simulink model "sampleModel1488"  (R2023a)
settings: Solver=VariableStepAuto  StartTime=0.0  StopTime=10.0  RelTol=1e-3
undefined symbols (not defined in the file): b011101a, b0c8, bf87616c, DiscIntNeverNeededParam, Newton, Raphson
libraries: simulink x171, slpidlib x32, simulink_need_slupdate x2
(part 6 of 6)

== system sampleModel1488/cfblk166/cfblk10 ==
  cfblk1 : Inport
  cfblk13 : Inport  Port=2
  cfblk14 : Inport  Port=3
  cfblk15 : Inport  Port=4
  cfblk10 : PermuteDimensions
  cfblk11 : Rounding
  cfblk12 : Sum  Inputs=|++
  cfblk3 : slpidlib/PID Controller (2DOF)  Controller=PID  Form=Parallel  TimeDomain=Discrete-time  UseExternalTs=off  SampleTime=1  IntegratorMethod=Forward Euler  FilterMethod=Forward Euler  ControllerParametersSource=internal  P=1  I=1  UseKiTs=off  D=0  N=100  UseFilter=on  b=1  c=1  TunerSelectOption=Transfer Function Based (PID Tuner App)  InitialConditionSource=internal  InitialConditionForIntegrator=0  InitialConditionForFilter=0  DifferentiatorICPrevScaledInput=0  ExternalReset=none  TrackingMode=off  Kt=1  LimitOutput=off  SatLimitsSource=internal  UpperSaturationLimit=inf  LowerSaturationLimit=-inf  LinearizeAsGain=off  AntiWindupMode=none  Kb=1  LimitIntegrator=off  UpperIntegratorSaturationLimit=inf  LowerIntegratorSaturationLimit=-inf  POutMin=[]  POutMax=[]  IOutMin=[]  IOutMax=[]  DOutMin=[]  DOutMax=[]  NOutMin=[]  NOutMax=[]  bOutMin=[]  bOutMax=[]  cOutMin=[]  cOutMax=[]  SumOutMin=[]  SumOutMax=[]  SaturationOutMin=[]  SaturationOutMax=[]  PParamMin=[]  PParamMax=[]  IParamMin=[]  IParamMax=[]  DParamMin=[]  DParamMax=[]  NParamMin=[]  NParamMax=[]  bParamMin=[]  bParamMax=[]  cParamMin=[]  cParamMax=[]  KbParamMin=[]  KbParamMax=[]  KtParamMin=[]  KtParamMax=[]  KbOutMin=[]  KbOutMax=[]  KtOutMin=[]  KtOutMax=[]  IntegratorOutMin=[]  IntegratorOutMax=[]  FilterOutMin=[]  FilterOutMax=[]  SumI1OutMin=[]  SumI1OutMax=[]  SumI2OutMin=[]  SumI2OutMax=[]  SumI3OutMin=[]  SumI3OutMax=[]  SumI4OutMin=[]  SumI4OutMax=[]  SumDOutMin=[]  SumDOutMax=[]  Sum1OutMin=[]  Sum1OutMax=[]  Sum2OutMin=[]  Sum2OutMax=[]  Sum3OutMin=[]  Sum3OutMax=[]  DifferentiatorOutMin=[]  DifferentiatorOutMax=[]  FilterDiffOutCoefMin=[]  FilterDiffOutCoefMax=[]  ReciprocalOutMin=[]  ReciprocalOutMax=[]  SumDenOutMin=[]  SumDenOutMax=[]  SumNumOutMin=[]  SumNumOutMax=[]  DivideOutMin=[]  DivideOutMax=[]  UdiffTsProdOutMin=[]  UdiffTsProdOutMax=[]  NTsProdOutMin=[]  NTsProdOutMax=[]  UintegralTsProdOutMin=[]  UintegralTsProdOutMax=[]  UngainTsProdOutMin=[]  UngainTsProdOutMax=[]  ClampingZeroOutDataTypeStr=Inherit: Inherit via back propagation  ClampingZeroOutMin=[]  ClampingZeroOutMax=[]  FilterDenConstantOutDataTypeStr=Inherit: Inherit via back propagation  FilterDenConstantOutMin=[]  FilterDenConstantOutMax=[]  PCopyOutDataTypeStr=Inherit: Inherit via back propagation  PCopyOutMin=[]  PCopyOutMax=[]  NCopyOutDataTypeStr=Inherit: Inherit via back propagation  NCopyOutMin=[]  NCopyOutMax=[]  IntegratorContinuousStateAttributes=''  IntegratorStateMustResolveToSignalObject=off  IntegratorRTWStateStorageClass=Auto  FilterContinuousStateAttributes=''  FilterStateMustResolveToSignalObject=off  FilterRTWStateStorageClass=Auto  ParallelPVariant=InternalParameters  IdealPVariant=Disabled  IVariant=InternalParameters  DVariant=InternalParameters  bVariant=InternalParameters  cVariant=InternalParameters  IntegratorVariant=Discrete  SatVariant=Disabled  AWVariant=Passthrough  PCopyVariant=Disabled  TRVariant=Disabled  FdbkBlocksVariant=Forward  IdealPFdbkVariant=Disabled  SatFdbkVariant=Disabled  DerivativeFilterVariant=ForwardEulerFilter  NVariant=InternalParameters  NCopyVariant=Disabled  FilterICVariant=InternalICsFilter  IntegratorICVariant=InternalICs  ExternalResetVariant=Disabled  TRSumVariant=Passthrough  SumFdbkVariant=Disabled  SumVariant=Sum_PID  TsampFilterVariant=InternalTs  TsampNgainVariant=Passthrough  TsampIntegralVariant=Disabled_SignalSpec  ExternalSaturationOutDataTypeStr=Inherit: Same as second input
      settings: LibrarySourceBlock=simulink/Discrete/Discrete PID Controller (2DOF)
  cfblk4 : DiscreteZeroPole  Poles=[0 0.5]  Gain=1
  cfblk5 : DiscreteZeroPole  Poles=[0 0.5]  Gain=1
  cfblk6 : slpidlib/PID Controller  Controller=PID  Form=Parallel  TimeDomain=Discrete-time  UseExternalTs=off  SampleTime=1  IntegratorMethod=Forward Euler  FilterMethod=Forward Euler  ControllerParametersSource=internal  P=1  I=1  UseKiTs=off  D=0  N=100  UseFilter=on  TunerSelectOption=Transfer Function Based (PID Tuner App)  InitialConditionSource=internal  InitialConditionForIntegrator=0  InitialConditionForFilter=0  DifferentiatorICPrevScaledInput=0  ExternalReset=none  TrackingMode=off  Kt=1  LimitOutput=off  SatLimitsSource=internal  UpperSaturationLimit=inf  LowerSaturationLimit=-inf  LinearizeAsGain=off  AntiWindupMode=none  Kb=1  LimitIntegrator=off  UpperIntegratorSaturationLimit=inf  LowerIntegratorSaturationLimit=-inf  POutMin=[]  POutMax=[]  IOutMin=[]  IOutMax=[]  DOutMin=[]  DOutMax=[]  NOutMin=[]  NOutMax=[]  SumOutMin=[]  SumOutMax=[]  SaturationOutMin=[]  SaturationOutMax=[]  PParamMin=[]  PParamMax=[]  IParamMin=[]  IParamMax=[]  DParamMin=[]  DParamMax=[]  NParamMin=[]  NParamMax=[]  KbParamMin=[]  KbParamMax=[]  KtParamMin=[]  KtParamMax=[]  KbOutMin=[]  KbOutMax=[]  KtOutMin=[]  KtOutMax=[]  IntegratorOutMin=[]  IntegratorOutMax=[]  FilterOutMin=[]  FilterOutMax=[]  SumI1OutMin=[]  SumI1OutMax=[]  SumI2OutMin=[]  SumI2OutMax=[]  SumI3OutMin=[]  SumI3OutMax=[]  SumI4OutMin=[]  SumI4OutMax=[]  SumDOutMin=[]  SumDOutMax=[]  DifferentiatorOutMin=[]  DifferentiatorOutMax=[]  FilterDiffOutCoefMin=[]  FilterDiffOutCoefMax=[]  ReciprocalOutMin=[]  ReciprocalOutMax=[]  SumDenOutMin=[]  SumDenOutMax=[]  SumNumOutMin=[]  SumNumOutMax=[]  DivideOutMin=[]  DivideOutMax=[]  UdiffTsProdOutMin=[]  UdiffTsProdOutMax=[]  NTsProdOutMin=[]  NTsProdOutMax=[]  UintegralTsProdOutMin=[]  UintegralTsProdOutMax=[]  UngainTsProdOutMin=[]  UngainTsProdOutMax=[]  ClampingZeroOutDataTypeStr=Inherit: Inherit via back propagation  ClampingZeroOutMin=[]  ClampingZeroOutMax=[]  FilterDenConstantOutDataTypeStr=Inherit: Inherit via back propagation  FilterDenConstantOutMin=[]  FilterDenConstantOutMax=[]  PCopyOutDataTypeStr=Inherit: Inherit via back propagation  PCopyOutMin=[]  PCopyOutMax=[]  NCopyOutDataTypeStr=Inherit: Inherit via back propagation  NCopyOutMin=[]  NCopyOutMax=[]  IntegratorContinuousStateAttributes=''  IntegratorStateMustResolveToSignalObject=off  IntegratorRTWStateStorageClass=Auto  FilterContinuousStateAttributes=''  FilterStateMustResolveToSignalObject=off  FilterRTWStateStorageClass=Auto  ParallelPVariant=InternalParameters  IdealPVariant=Disabled  IVariant=InternalParameters  DVariant=InternalParameters  IntegratorVariant=Discrete  SatVariant=Disabled  AWVariant=Passthrough  PCopyVariant=Disabled  TRVariant=Disabled  FdbkBlocksVariant=Forward  IdealPFdbkVariant=Disabled  SatFdbkVariant=Disabled  DerivativeFilterVariant=ForwardEulerFilter  NVariant=InternalParameters  NCopyVariant=Disabled  FilterICVariant=InternalICsFilter  IntegratorICVariant=InternalICs  ExternalResetVariant=Disabled  TRSumVariant=Passthrough  SumFdbkVariant=Disabled  SumVariant=Sum_PID  TsampFilterVariant=InternalTs  TsampNgainVariant=Passthrough  TsampIntegralVariant=Disabled_SignalSpec  ExternalSaturationOutDataTypeStr=Inherit: Same as second input
      settings: LibrarySourceBlock=simulink/Discrete/Discrete PID Controller
  cfblk7 : MinMax  Function=max  Inputs=2
  cfblk8 : Sqrt  Operator=rSqrt  AlgorithmType=Newton-Raphson
  cfblk9 : Sum  Inputs=+-
  cfblk2 : Outport
  cfblk16 : Outport  Port=2
  cfblk17 : Outport  Port=3
  wires:
  cfblk5/1 -> cfblk2/1
  cfblk9/1 -> cfblk3/1
  cfblk8/1 -> cfblk7/1
  cfblk4/1 -> cfblk8/1
  cfblk13/1 -> cfblk3/2, cfblk12/2
  cfblk6/1 -> cfblk10/1
  cfblk14/1 -> cfblk11/1
  cfblk3/1 -> cfblk7/2
  cfblk11/1 -> cfblk4/1, cfblk12/1
  cfblk7/1 -> cfblk5/1, cfblk17/1
  cfblk1/1 -> cfblk16/1
  cfblk15/1 -> cfblk9/1
  cfblk12/1 -> cfblk6/1
  cfblk10/1 -> cfblk9/2

== system sampleModel1488/cfblk166/cfblk11 ==
  cfblk1 : Inport
  cfblk10 : Inport  Port=2
  cfblk11 : Inport  Port=3
  cfblk12 : Inport  Port=4
  cfblk13 : Inport  Port=5
  cfblk3 : simulink/Discrete/Transfer Fcn Lead or Lag  PoleZ=0.95  ZeroZ=0.75  ICPrevOutput=0.0  ICPrevInput=0.0  DoSatur=off
  cfblk4 : Rounding
  cfblk5 : Assignment  DiagnosticForDimensions=Warning  IndexOptions=Index vector (dialog)  Indices=1  OutputSizes=1
  cfblk6 : Signum
  cfblk7 : Constant  Value=[402326057.217924]  SampleTime=1
  cfblk8 : Constant  Value=[-430867687.109002]  SampleTime=1
  cfblk9 : Constant  Value=[874146926.487042]  SampleTime=1
  cfblk2 : Outport
  wires:
  cfblk3/1 -> cfblk2/1
  cfblk9/1 -> cfblk3/1
  cfblk10/1 -> cfblk5/1
  cfblk4/1 -> cfblk6/1
  cfblk6/1 -> cfblk5/2
  cfblk7/1 -> cfblk4/1

== system sampleModel1488/cfblk166/cfblk9 ==
  cfblk1 : Inport
  cfblk11 : Inport  Port=2
  cfblk12 : Inport  Port=3
  cfblk13 : Inport  Port=4
  cfblk14 : Inport  Port=5
  cfblk10 : Constant  Value=[-771361582.473640]  SampleTime=1
  cfblk3 : DiscreteTransferFcn  SampleTime=1
  cfblk4 : Bias  Bias=[-976022040.678061]  SaturateOnIntegerOverflow=off
  cfblk5 : ComplexToMagnitudeAngle
  cfblk6 : Sqrt
  cfblk7 : Math  Operator=hypot
  cfblk8 : Constant  Value=[35530573.670339]  SampleTime=1
  cfblk9 : Constant  Value=[264514942.100950]  SampleTime=1
  cfblk2 : Outport
  cfblk15 : Outport  Port=2
  wires:
  cfblk6/1 -> cfblk5/1
  cfblk9/1 -> cfblk2/1
  cfblk8/1 -> cfblk4/1
  cfblk13/1 -> cfblk6/1
  cfblk3/1 -> cfblk7/1
  cfblk4/1 -> cfblk7/2
  cfblk14/1 -> cfblk15/1
  cfblk11/1 -> cfblk3/1

== system sampleModel1488/cfblk167/cfblk10 ==
  cfblk1 : Inport
  cfblk8 : Inport  Port=2
  cfblk3 : simulink/Discrete/Tapped Delay  vinit=0.0  samptime=-1  NumDelays=1  DelayOrder=Oldest  includeCurrent=off
  cfblk4 : DiscreteTransferFcn  SampleTime=1
  cfblk5 : DiscreteFilter  SampleTime=1
  cfblk6 : ComplexToMagnitudeAngle
  cfblk7 : simulink/Math Operations/Slider Gain  gain=1  low=0  high=2
  cfblk9 : Delay  SampleTime=1
  cfblk2 : Outport
  wires:
  cfblk1/1 -> cfblk4/1
  cfblk8/1 -> cfblk2/1
  cfblk4/1 -> cfblk3/1
  cfblk6/1 -> cfblk7/1
  cfblk5/1 -> cfblk6/1
  cfblk6/2 -> cfblk9/1
  cfblk9/1 -> cfblk5/1

== system sampleModel1488/cfblk167/cfblk11 ==
  cfblk1 : Inport
  cfblk8 : Inport  Port=2
  cfblk3 : simulink/Discrete/Difference  ICPrevInput=0.0  OutMin=[]  OutMax=[]  OutDataTypeStr=Inherit: Inherit via back propagation  OutDataType=fixdt(1, 16)  OutScaling=2^-10  DoSatur=off
  cfblk4 : DotProduct  OutDataTypeStr=Inherit: Inherit via internal rule
  cfblk5 : Product
  cfblk6 : MinMax  Function=max  Inputs=3
  cfblk7 : Constant  Value=[-875675673.785562]  SampleTime=1
  cfblk2 : Outport
  cfblk9 : Outport  Port=2
  wires:
  cfblk6/1 -> cfblk2/1
  cfblk1/1 -> cfblk5/1, cfblk6/3
  cfblk5/1 -> cfblk3/1
  cfblk7/1 -> cfblk5/2, cfblk4/2
  cfblk4/1 -> cfblk9/1
  cfblk3/1 -> cfblk6/1, cfblk6/2
  cfblk8/1 -> cfblk4/1

== system sampleModel1488/cfblk167/cfblk12 ==
  cfblk1 : Inport
  cfblk10 : Constant  Value=[-895011332.813341]  SampleTime=1
  cfblk11 : Constant  Value=[842655779.638818]  SampleTime=1
  cfblk13 : Delay  SampleTime=1
  cfblk3 : DiscreteTransferFcn  SampleTime=1
  cfblk4 : Delay  ShowEnablePort=on  SampleTime=1
      settings: InputPortMap=u0,e6
  cfblk5 : slpidlib/PID Controller  Controller=PID  Form=Parallel  TimeDomain=Discrete-time  UseExternalTs=off  SampleTime=1  IntegratorMethod=Forward Euler  FilterMethod=Forward Euler  ControllerParametersSource=internal  P=1  I=1  UseKiTs=off  D=0  N=100  UseFilter=on  TunerSelectOption=Transfer Function Based (PID Tuner App)  InitialConditionSource=internal  InitialConditionForIntegrator=0  InitialConditionForFilter=0  DifferentiatorICPrevScaledInput=0  ExternalReset=none  TrackingMode=off  Kt=1  LimitOutput=off  SatLimitsSource=internal  UpperSaturationLimit=inf  LowerSaturationLimit=-inf  LinearizeAsGain=off  AntiWindupMode=none  Kb=1  LimitIntegrator=off  UpperIntegratorSaturationLimit=inf  LowerIntegratorSaturationLimit=-inf  POutMin=[]  POutMax=[]  IOutMin=[]  IOutMax=[]  DOutMin=[]  DOutMax=[]  NOutMin=[]  NOutMax=[]  SumOutMin=[]  SumOutMax=[]  SaturationOutMin=[]  SaturationOutMax=[]  PParamMin=[]  PParamMax=[]  IParamMin=[]  IParamMax=[]  DParamMin=[]  DParamMax=[]  NParamMin=[]  NParamMax=[]  KbParamMin=[]  KbParamMax=[]  KtParamMin=[]  KtParamMax=[]  KbOutMin=[]  KbOutMax=[]  KtOutMin=[]  KtOutMax=[]  IntegratorOutMin=[]  IntegratorOutMax=[]  FilterOutMin=[]  FilterOutMax=[]  SumI1OutMin=[]  SumI1OutMax=[]  SumI2OutMin=[]  SumI2OutMax=[]  SumI3OutMin=[]  SumI3OutMax=[]  SumI4OutMin=[]  SumI4OutMax=[]  SumDOutMin=[]  SumDOutMax=[]  DifferentiatorOutMin=[]  DifferentiatorOutMax=[]  FilterDiffOutCoefMin=[]  FilterDiffOutCoefMax=[]  ReciprocalOutMin=[]  ReciprocalOutMax=[]  SumDenOutMin=[]  SumDenOutMax=[]  SumNumOutMin=[]  SumNumOutMax=[]  DivideOutMin=[]  DivideOutMax=[]  UdiffTsProdOutMin=[]  UdiffTsProdOutMax=[]  NTsProdOutMin=[]  NTsProdOutMax=[]  UintegralTsProdOutMin=[]  UintegralTsProdOutMax=[]  UngainTsProdOutMin=[]  UngainTsProdOutMax=[]  ClampingZeroOutDataTypeStr=Inherit: Inherit via back propagation  ClampingZeroOutMin=[]  ClampingZeroOutMax=[]  FilterDenConstantOutDataTypeStr=Inherit: Inherit via back propagation  FilterDenConstantOutMin=[]  FilterDenConstantOutMax=[]  PCopyOutDataTypeStr=Inherit: Inherit via back propagation  PCopyOutMin=[]  PCopyOutMax=[]  NCopyOutDataTypeStr=Inherit: Inherit via back propagation  NCopyOutMin=[]  NCopyOutMax=[]  IntegratorContinuousStateAttributes=''  IntegratorStateMustResolveToSignalObject=off  IntegratorRTWStateStorageClass=Auto  FilterContinuousStateAttributes=''  FilterStateMustResolveToSignalObject=off  FilterRTWStateStorageClass=Auto  ParallelPVariant=InternalParameters  IdealPVariant=Disabled  IVariant=InternalParameters  DVariant=InternalParameters  IntegratorVariant=Discrete  SatVariant=Disabled  AWVariant=Passthrough  PCopyVariant=Disabled  TRVariant=Disabled  FdbkBlocksVariant=Forward  IdealPFdbkVariant=Disabled  SatFdbkVariant=Disabled  DerivativeFilterVariant=ForwardEulerFilter  NVariant=InternalParameters  NCopyVariant=Disabled  FilterICVariant=InternalICsFilter  IntegratorICVariant=InternalICs  ExternalResetVariant=Disabled  TRSumVariant=Passthrough  SumFdbkVariant=Disabled  SumVariant=Sum_PID  TsampFilterVariant=InternalTs  TsampNgainVariant=Passthrough  TsampIntegralVariant=Disabled_SignalSpec  ExternalSaturationOutDataTypeStr=Inherit: Same as second input
      settings: LibrarySourceBlock=simulink/Discrete/Discrete PID Controller
  cfblk6 : Product
  cfblk7 : simulink/Math Operations/Slider Gain  gain=1  low=0  high=2
  cfblk8 : simulink/Math Operations/Slider Gain  gain=1  low=0  high=2
  cfblk9 : Signum
  cfblk2 : Outport
  cfblk12 : Outport  Port=2
  wires:
  cfblk9/1 -> cfblk4/1
  cfblk4/1 -> cfblk2/1
  cfblk3/1 -> cfblk5/1
  cfblk11/1 -> cfblk9/1
  cfblk10/1 -> cfblk3/1
  cfblk6/1 -> cfblk7/1
  cfblk7/1 -> cfblk8/1, cfblk13/1
  cfblk1/1 -> cfblk4/2
  cfblk5/1 -> cfblk6/1
  cfblk8/1 -> cfblk12/1
  cfblk13/1 -> cfblk6/2

== system sampleModel1488/cfblk168/cfblk8 ==
  cfblk1 : Inport
  cfblk8 : Inport  Port=2
  cfblk9 : Inport  Port=3
  cfblk10 : Inport  Port=4
  cfblk11 : Inport  Port=5
  cfblk12 : Inport  Port=6
  cfblk3 : DiscreteTransferFcn  SampleTime=1
  cfblk4 : simulink/Math Operations/Slider Gain  gain=1  low=0  high=2
  cfblk5 : Assignment  DiagnosticForDimensions=Warning  IndexOptions=Index vector (dialog)  Indices=1  OutputSizes=1
  cfblk6 : Constant  Value=[866048568.581870]  SampleTime=1
  cfblk7 : Constant  Value=[-416368568.572532]  SampleTime=1
  cfblk2 : Outport
  cfblk13 : Outport  Port=2
  cfblk14 : Outport  Port=3
  cfblk15 : Outport  Port=4
  wires:
  cfblk11/1 -> cfblk14/1
  cfblk8/1 -> cfblk2/1
  cfblk7/1 -> cfblk15/1
  cfblk12/1 -> cfblk5/1
  cfblk1/1 -> cfblk3/1
  cfblk3/1 -> cfblk13/1
  cfblk6/1 -> cfblk5/2
  cfblk5/1 -> cfblk4/1

== system sampleModel1488/cfblk169/cfblk6 ==
  cfblk1 : Inport
  cfblk10 : Squeeze
  cfblk11 : Gain  Gain=[654237214.997808]
  cfblk12 : Sqrt  Operator=rSqrt  AlgorithmType=Newton-Raphson
  cfblk13 : Constant  Value=[855856144.251508]  SampleTime=1
  cfblk15 : Delay  SampleTime=1
  cfblk16 : Delay  SampleTime=1
  cfblk3 : simulink/Discrete/Transfer Fcn Lead or Lag  PoleZ=0.95  ZeroZ=0.75  ICPrevOutput=0.0  ICPrevInput=0.0  DoSatur=off
  cfblk4 : Delay  SampleTime=1
  cfblk5 : simulink/Discrete/Transfer Fcn Real Zero  ZeroZ=0.75  ICPrevInput=0.0  DoSatur=off
  cfblk6 : DiscreteStateSpace
  cfblk7 : slpidlib/PID Controller (2DOF)  Controller=PID  Form=Parallel  TimeDomain=Discrete-time  UseExternalTs=off  SampleTime=1  IntegratorMethod=Forward Euler  FilterMethod=Forward Euler  ControllerParametersSource=internal  P=1  I=1  UseKiTs=off  D=0  N=100  UseFilter=on  b=1  c=1  TunerSelectOption=Transfer Function Based (PID Tuner App)  InitialConditionSource=internal  InitialConditionForIntegrator=0  InitialConditionForFilter=0  DifferentiatorICPrevScaledInput=0  ExternalReset=none  TrackingMode=off  Kt=1  LimitOutput=off  SatLimitsSource=internal  UpperSaturationLimit=inf  LowerSaturationLimit=-inf  LinearizeAsGain=off  AntiWindupMode=none  Kb=1  LimitIntegrator=off  UpperIntegratorSaturationLimit=inf  LowerIntegratorSaturationLimit=-inf  POutMin=[]  POutMax=[]  IOutMin=[]  IOutMax=[]  DOutMin=[]  DOutMax=[]  NOutMin=[]  NOutMax=[]  bOutMin=[]  bOutMax=[]  cOutMin=[]  cOutMax=[]  SumOutMin=[]  SumOutMax=[]  SaturationOutMin=[]  SaturationOutMax=[]  PParamMin=[]  PParamMax=[]  IParamMin=[]  IParamMax=[]  DParamMin=[]  DParamMax=[]  NParamMin=[]  NParamMax=[]  bParamMin=[]  bParamMax=[]  cParamMin=[]  cParamMax=[]  KbParamMin=[]  KbParamMax=[]  KtParamMin=[]  KtParamMax=[]  KbOutMin=[]  KbOutMax=[]  KtOutMin=[]  KtOutMax=[]  IntegratorOutMin=[]  IntegratorOutMax=[]  FilterOutMin=[]  FilterOutMax=[]  SumI1OutMin=[]  SumI1OutMax=[]  SumI2OutMin=[]  SumI2OutMax=[]  SumI3OutMin=[]  SumI3OutMax=[]  SumI4OutMin=[]  SumI4OutMax=[]  SumDOutMin=[]  SumDOutMax=[]  Sum1OutMin=[]  Sum1OutMax=[]  Sum2OutMin=[]  Sum2OutMax=[]  Sum3OutMin=[]  Sum3OutMax=[]  DifferentiatorOutMin=[]  DifferentiatorOutMax=[]  FilterDiffOutCoefMin=[]  FilterDiffOutCoefMax=[]  ReciprocalOutMin=[]  ReciprocalOutMax=[]  SumDenOutMin=[]  SumDenOutMax=[]  SumNumOutMin=[]  SumNumOutMax=[]  DivideOutMin=[]  DivideOutMax=[]  UdiffTsProdOutMin=[]  UdiffTsProdOutMax=[]  NTsProdOutMin=[]  NTsProdOutMax=[]  UintegralTsProdOutMin=[]  UintegralTsProdOutMax=[]  UngainTsProdOutMin=[]  UngainTsProdOutMax=[]  ClampingZeroOutDataTypeStr=Inherit: Inherit via back propagation  ClampingZeroOutMin=[]  ClampingZeroOutMax=[]  FilterDenConstantOutDataTypeStr=Inherit: Inherit via back propagation  FilterDenConstantOutMin=[]  FilterDenConstantOutMax=[]  PCopyOutDataTypeStr=Inherit: Inherit via back propagation  PCopyOutMin=[]  PCopyOutMax=[]  NCopyOutDataTypeStr=Inherit: Inherit via back propagation  NCopyOutMin=[]  NCopyOutMax=[]  IntegratorContinuousStateAttributes=''  IntegratorStateMustResolveToSignalObject=off  IntegratorRTWStateStorageClass=Auto  FilterContinuousStateAttributes=''  FilterStateMustResolveToSignalObject=off  FilterRTWStateStorageClass=Auto  ParallelPVariant=InternalParameters  IdealPVariant=Disabled  IVariant=InternalParameters  DVariant=InternalParameters  bVariant=InternalParameters  cVariant=InternalParameters  IntegratorVariant=Discrete  SatVariant=Disabled  AWVariant=Passthrough  PCopyVariant=Disabled  TRVariant=Disabled  FdbkBlocksVariant=Forward  IdealPFdbkVariant=Disabled  SatFdbkVariant=Disabled  DerivativeFilterVariant=ForwardEulerFilter  NVariant=InternalParameters  NCopyVariant=Disabled  FilterICVariant=InternalICsFilter  IntegratorICVariant=InternalICs  ExternalResetVariant=Disabled  TRSumVariant=Passthrough  SumFdbkVariant=Disabled  SumVariant=Sum_PID  TsampFilterVariant=InternalTs  TsampNgainVariant=Passthrough  TsampIntegralVariant=Disabled_SignalSpec  ExternalSaturationOutDataTypeStr=Inherit: Same as second input
      settings: LibrarySourceBlock=simulink/Discrete/Discrete PID Controller (2DOF)
  cfblk8 : Abs  SaturateOnIntegerOverflow=off
  cfblk9 : Abs  SaturateOnIntegerOverflow=off
  cfblk2 : Outport
  cfblk14 : Outport  Port=2
  wires:
  cfblk11/1 -> cfblk3/1
  cfblk6/1 -> cfblk10/1
  cfblk3/1 -> cfblk2/1
  cfblk1/1 -> cfblk12/1
  cfblk4/1 -> cfblk8/1
  cfblk13/1 -> cfblk11/1
  cfblk12/1 -> cfblk14/1
  cfblk9/1 -> cfblk6/1, cfblk5/1
  cfblk8/1 -> cfblk7/2
  cfblk7/1 -> cfblk9/1
  cfblk10/1 -> cfblk15/1
  cfblk15/1 -> cfblk7/1
  cfblk5/1 -> cfblk16/1
  cfblk16/1 -> cfblk4/1

== system sampleModel1488/cfblk169/cfblk7 ==
  cfblk1 : Inport
  cfblk10 : Math
  cfblk11 : ComplexToMagnitudeAngle
  cfblk12 : Abs  SaturateOnIntegerOverflow=off
  cfblk13 : Sin  TimeSource=Use external signal  SampleTime=0
  cfblk14 : Sum  Inputs=|++
  cfblk15 : Abs  SaturateOnIntegerOverflow=off
  cfblk16 : Constant  Value=[-144295758.611368]  SampleTime=1
  cfblk17 : Delay  SampleTime=1
  cfblk18 : Delay  SampleTime=1
  cfblk3 : PropagationDelay  SampleTime=1
  cfblk4 : slpidlib/PID Controller  Controller=PID  Form=Parallel  TimeDomain=Discrete-time  UseExternalTs=off  SampleTime=1  IntegratorMethod=Forward Euler  FilterMethod=Forward Euler  ControllerParametersSource=internal  P=1  I=1  UseKiTs=off  D=0  N=100  UseFilter=on  TunerSelectOption=Transfer Function Based (PID Tuner App)  InitialConditionSource=internal  InitialConditionForIntegrator=0  InitialConditionForFilter=0  DifferentiatorICPrevScaledInput=0  ExternalReset=none  TrackingMode=off  Kt=1  LimitOutput=off  SatLimitsSource=internal  UpperSaturationLimit=inf  LowerSaturationLimit=-inf  LinearizeAsGain=off  AntiWindupMode=none  Kb=1  LimitIntegrator=off  UpperIntegratorSaturationLimit=inf  LowerIntegratorSaturationLimit=-inf  POutMin=[]  POutMax=[]  IOutMin=[]  IOutMax=[]  DOutMin=[]  DOutMax=[]  NOutMin=[]  NOutMax=[]  SumOutMin=[]  SumOutMax=[]  SaturationOutMin=[]  SaturationOutMax=[]  PParamMin=[]  PParamMax=[]  IParamMin=[]  IParamMax=[]  DParamMin=[]  DParamMax=[]  NParamMin=[]  NParamMax=[]  KbParamMin=[]  KbParamMax=[]  KtParamMin=[]  KtParamMax=[]  KbOutMin=[]  KbOutMax=[]  KtOutMin=[]  KtOutMax=[]  IntegratorOutMin=[]  IntegratorOutMax=[]  FilterOutMin=[]  FilterOutMax=[]  SumI1OutMin=[]  SumI1OutMax=[]  SumI2OutMin=[]  SumI2OutMax=[]  SumI3OutMin=[]  SumI3OutMax=[]  SumI4OutMin=[]  SumI4OutMax=[]  SumDOutMin=[]  SumDOutMax=[]  DifferentiatorOutMin=[]  DifferentiatorOutMax=[]  FilterDiffOutCoefMin=[]  FilterDiffOutCoefMax=[]  ReciprocalOutMin=[]  ReciprocalOutMax=[]  SumDenOutMin=[]  SumDenOutMax=[]  SumNumOutMin=[]  SumNumOutMax=[]  DivideOutMin=[]  DivideOutMax=[]  UdiffTsProdOutMin=[]  UdiffTsProdOutMax=[]  NTsProdOutMin=[]  NTsProdOutMax=[]  UintegralTsProdOutMin=[]  UintegralTsProdOutMax=[]  UngainTsProdOutMin=[]  UngainTsProdOutMax=[]  ClampingZeroOutDataTypeStr=Inherit: Inherit via back propagation  ClampingZeroOutMin=[]  ClampingZeroOutMax=[]  FilterDenConstantOutDataTypeStr=Inherit: Inherit via back propagation  FilterDenConstantOutMin=[]  FilterDenConstantOutMax=[]  PCopyOutDataTypeStr=Inherit: Inherit via back propagation  PCopyOutMin=[]  PCopyOutMax=[]  NCopyOutDataTypeStr=Inherit: Inherit via back propagation  NCopyOutMin=[]  NCopyOutMax=[]  IntegratorContinuousStateAttributes=''  IntegratorStateMustResolveToSignalObject=off  IntegratorRTWStateStorageClass=Auto  FilterContinuousStateAttributes=''  FilterStateMustResolveToSignalObject=off  FilterRTWStateStorageClass=Auto  ParallelPVariant=InternalParameters  IdealPVariant=Disabled  IVariant=InternalParameters  DVariant=InternalParameters  IntegratorVariant=Discrete  SatVariant=Disabled  AWVariant=Passthrough  PCopyVariant=Disabled  TRVariant=Disabled  FdbkBlocksVariant=Forward  IdealPFdbkVariant=Disabled  SatFdbkVariant=Disabled  DerivativeFilterVariant=ForwardEulerFilter  NVariant=InternalParameters  NCopyVariant=Disabled  FilterICVariant=InternalICsFilter  IntegratorICVariant=InternalICs  ExternalResetVariant=Disabled  TRSumVariant=Passthrough  SumFdbkVariant=Disabled  SumVariant=Sum_PID  TsampFilterVariant=InternalTs  TsampNgainVariant=Passthrough  TsampIntegralVariant=Disabled_SignalSpec  ExternalSaturationOutDataTypeStr=Inherit: Same as second input
      settings: LibrarySourceBlock=simulink/Discrete/Discrete PID Controller
  cfblk5 : Rounding
  cfblk6 : Sum  Inputs=+
  cfblk7 : Math  Operator=conj
  cfblk8 : Polyval  Coefs=[ +2.081618890e-019, -1.441693666e-014, +4.719686976e-010, -8.536869453e-006, +1.621573104e-001, -8.087801117e+001 ]
  cfblk9 : UnaryMinus
  cfblk2 : Outport
  wires:
  cfblk12/1 -> cfblk8/1
  cfblk4/1 -> cfblk9/1
  cfblk9/1 -> cfblk12/1
  cfblk15/1 -> cfblk10/1
  cfblk16/1 -> cfblk14/1
  cfblk7/1 -> cfblk11/1
  cfblk5/1 -> cfblk15/1
  cfblk3/1 -> cfblk6/1
  cfblk1/1 -> cfblk3/2
  cfblk14/1 -> cfblk13/1
  cfblk13/1 -> cfblk5/1
  cfblk8/1 -> cfblk14/2
  cfblk11/2 -> cfblk2/1
  cfblk6/1 -> cfblk4/1
  cfblk10/1 -> cfblk17/1
  cfblk17/1 -> cfblk3/1
  cfblk11/1 -> cfblk18/1
  cfblk18/1 -> cfblk7/1

== system sampleModel1488/cfblk169/cfblk8 ==
  cfblk1 : Inport
  cfblk3 : DiscreteZeroPole  Poles=[0 0.5]  Gain=1
  cfblk4 : Rounding
  cfblk5 : Sum  Inputs=+-
  cfblk6 : Constant  Value=[834853285.484630]  SampleTime=1
  cfblk2 : Outport
  cfblk7 : Outport  Port=2
  wires:
  cfblk3/1 -> cfblk2/1
  cfblk5/1 -> cfblk3/1
  cfblk1/1 -> cfblk4/1
  cfblk4/1 -> cfblk5/1, cfblk7/1
  cfblk6/1 -> cfblk5/2

== system sampleModel1488/cfblk170/cfblk10 ==
  cfblk1 : Inport
  cfblk10 : Inport  Port=2
  cfblk11 : Inport  Port=3
  cfblk3 : DiscreteTransferFcn  SampleTime=1
  cfblk4 : simulink/Discrete/Transfer Fcn Real Zero  ZeroZ=0.75  ICPrevInput=0.0  DoSatur=off
  cfblk5 : MinMax  Inputs=2
  cfblk6 : simulink/Math Operations/MinMax Running Resettable  Function=min  vinit=0.0
  cfblk7 : Abs  SaturateOnIntegerOverflow=off
  cfblk8 : Assignment  DiagnosticForDimensions=Warning  IndexOptions=Index vector (dialog)  Indices=1  OutputSizes=1
  cfblk9 : Constant  Value=[424288837.357082]  SampleTime=1
  cfblk2 : Outport
  wires:
  cfblk11/1 -> cfblk6/1
  cfblk1/1 -> cfblk3/1
  cfblk3/1 -> cfblk5/1
  cfblk8/1 -> cfblk4/1
  cfblk9/1 -> cfblk8/1
  cfblk7/1 -> cfblk2/1
  cfblk5/1 -> cfblk8/2
  cfblk6/1 -> cfblk5/2
  cfblk4/1 -> cfblk7/1
  cfblk10/1 -> cfblk6/2

== system sampleModel1488/cfblk170/cfblk12 ==
  cfblk1 : Inport
  cfblk12 : Inport  Port=2
  cfblk13 : Inport  Port=3
  cfblk14 : Inport  Port=4
  cfblk15 : Inport  Port=5
  Action Port : ActionPort  ActionPortLabel=if(u1 >= 0)
  cfblk10 : Gain  Gain=[-219968624.405801]
  cfblk11 : ComplexToMagnitudeAngle
  cfblk3 : DiscreteFilter
  cfblk4 : DiscreteFilter
  cfblk5 : DiscreteIntegrator  SampleTime=-1  ICPrevOutput=DiscIntNeverNeededParam  ICPrevScaledInput=DiscIntNeverNeededParam
  cfblk6 : Delay
  cfblk7 : PermuteDimensions
  cfblk8 : Sum  Inputs=|++
  cfblk9 : Product  Inputs=**
  cfblk2 : Outport
  wires:
  cfblk13/1 -> cfblk9/1
  cfblk9/1 -> cfblk11/1
  cfblk1/1 -> cfblk5/1
  cfblk6/1 -> cfblk2/1
  cfblk11/1 -> cfblk10/1
  cfblk7/1 -> cfblk6/1
  cfblk4/1 -> cfblk3/1
  cfblk10/1 -> cfblk4/1
  cfblk14/1 -> cfblk8/1
  cfblk12/1 -> cfblk8/2
  cfblk11/2 -> cfblk7/1
  cfblk8/1 -> cfblk9/2

== system sampleModel1488/cfblk170/cfblk13 ==
  cfblk1 : Inport
  cfblk7 : Inport  Port=2
  cfblk8 : Inport  Port=3
  Action Port : ActionPort  ActionPortLabel=else
  cfblk3 : Delay  ShowEnablePort=on
      settings: InputPortMap=u0,e6
  cfblk4 : Rounding
  cfblk5 : PermuteDimensions
  cfblk6 : Polyval  Coefs=[ +2.081618890e-019, -1.441693666e-014, +4.719686976e-010, -8.536869453e-006, +1.621573104e-001, -8.087801117e+001 ]
  cfblk2 : Outport
  cfblk9 : Outport  Port=2
  wires:
  cfblk8/1 -> cfblk2/1
  cfblk4/1 -> cfblk9/1
  cfblk3/1 -> cfblk4/1
  cfblk7/1 -> cfblk5/1
  cfblk5/1 -> cfblk6/1
  cfblk1/1 -> cfblk3/1
  cfblk6/1 -> cfblk3/2

== system sampleModel1488/cfblk171/cfblk6 ==
  cfblk1 : Inport
  cfblk11 : Inport  Port=2
  cfblk12 : Inport  Port=3
  cfblk13 : Inport  Port=4
  cfblk10 : Constant  Value=[520548367.549841]  SampleTime=1
  cfblk3 : UnitDelay  HasFrameUpgradeWarning=on
  cfblk4 : Sum  Inputs=+-
  cfblk5 : Sin  TimeSource=Use external signal  SampleTime=0
  cfblk6 : ComplexToRealImag
  cfblk7 : Abs  SaturateOnIntegerOverflow=off
  cfblk8 : ComplexToMagnitudeAngle
  cfblk9 : Sum  Inputs=+
  cfblk2 : Outport
  cfblk14 : Outport  Port=2
  wires:
  cfblk11/1 -> cfblk3/1
  cfblk8/1 -> cfblk5/1
  cfblk1/1 -> cfblk8/1
  cfblk8/2 -> cfblk6/1
  cfblk7/1 -> cfblk9/1
  cfblk3/1 -> cfblk7/1
  cfblk13/1 -> cfblk14/1
  cfblk4/1 -> cfblk2/1
  cfblk12/1 -> cfblk4/1
  cfblk10/1 -> cfblk4/2

== system sampleModel1488/cfblk171/cfblk7 ==
  cfblk1 : Inport
  cfblk7 : Inport  Port=2
  cfblk8 : Inport  Port=3
  cfblk10 : Delay  SampleTime=1
  cfblk3 : DiscreteZeroPole  Poles=[0 0.5]  Gain=1
  cfblk4 : simulink/Math Operations/Slider Gain  gain=1  low=0  high=2
  cfblk5 : ComplexToMagnitudeAngle
  cfblk6 : Product  Inputs=**
  cfblk2 : Outport
  cfblk9 : Outport  Port=2
  wires:
  cfblk7/1 -> cfblk2/1
  cfblk8/1 -> cfblk4/1
  cfblk1/1 -> cfblk9/1
  cfblk4/1 -> cfblk5/1
  cfblk5/1 -> cfblk6/1
  cfblk3/1 -> cfblk6/2
  cfblk6/1 -> cfblk10/1
  cfblk10/1 -> cfblk3/1

== system sampleModel1488/cfblk172/cfblk10 ==
  cfblk1 : Inport
  cfblk8 : Inport  Port=2
  cfblk9 : Inport  Port=3
  cfblk10 : Delay  SampleTime=1
  cfblk3 : simulink/Discrete/Transfer Fcn Lead or Lag  PoleZ=0.95  ZeroZ=0.75  ICPrevOutput=0.0  ICPrevInput=0.0  DoSatur=off
  cfblk4 : DiscreteFilter  SampleTime=1
  cfblk5 : MinMax  Inputs=3
  cfblk6 : DotProduct  OutDataTypeStr=Inherit: Inherit via internal rule
  cfblk7 : Product  Inputs=**
  cfblk2 : Outport
  wires:
  cfblk4/1 -> cfblk7/1
  cfblk7/1 -> cfblk5/1
  cfblk6/1 -> cfblk7/2
  cfblk9/1 -> cfblk5/2
  cfblk3/1 -> cfblk5/3
  cfblk8/1 -> cfblk3/1
  cfblk5/1 -> cfblk2/1, cfblk10/1
  cfblk1/1 -> cfblk6/2, cfblk4/1
  cfblk10/1 -> cfblk6/1

== system sampleModel1488/cfblk172/cfblk11 ==
  cfblk1 : Inport
  cfblk7 : Inport  Port=2
  cfblk8 : Inport  Port=3
  cfblk3 : simulink/Discrete/Transfer Fcn Real Zero  ZeroZ=0.75  ICPrevInput=0.0  DoSatur=off
  cfblk4 : Trigonometry
  cfblk5 : PermuteDimensions
  cfblk6 : Constant  Value=[-437669265.205893]  SampleTime=1
  cfblk2 : Outport
  wires:
  cfblk8/1 -> cfblk5/1
  cfblk4/1 -> cfblk2/1
  cfblk5/1 -> cfblk4/1
  cfblk1/1 -> cfblk3/1

== system sampleModel1488/cfblk172/cfblk12 ==
  cfblk1 : Inport
  cfblk14 : Inport  Port=2
  cfblk15 : Inport  Port=3
  cfblk16 : Inport  Port=4
  cfblk10 : MinMax  Inputs=3
  cfblk11 : Constant  Value=[-593358333.557490]  SampleTime=1
  cfblk12 : Constant  Value=[-613940772.920416]  SampleTime=1
  cfblk13 : Constant  Value=[-836179113.177943]  SampleTime=1
  cfblk3 : slpidlib/PID Controller (2DOF)  Controller=PID  Form=Parallel  TimeDomain=Discrete-time  UseExternalTs=off  SampleTime=1  IntegratorMethod=Forward Euler  FilterMethod=Forward Euler  ControllerParametersSource=internal  P=1  I=1  UseKiTs=off  D=0  N=100  UseFilter=on  b=1  c=1  TunerSelectOption=Transfer Function Based (PID Tuner App)  InitialConditionSource=internal  InitialConditionForIntegrator=0  InitialConditionForFilter=0  DifferentiatorICPrevScaledInput=0  ExternalReset=none  TrackingMode=off  Kt=1  LimitOutput=off  SatLimitsSource=internal  UpperSaturationLimit=inf  LowerSaturationLimit=-inf  LinearizeAsGain=off  AntiWindupMode=none  Kb=1  LimitIntegrator=off  UpperIntegratorSaturationLimit=inf  LowerIntegratorSaturationLimit=-inf  POutMin=[]  POutMax=[]  IOutMin=[]  IOutMax=[]  DOutMin=[]  DOutMax=[]  NOutMin=[]  NOutMax=[]  bOutMin=[]  bOutMax=[]  cOutMin=[]  cOutMax=[]  SumOutMin=[]  SumOutMax=[]  SaturationOutMin=[]  SaturationOutMax=[]  PParamMin=[]  PParamMax=[]  IParamMin=[]  IParamMax=[]  DParamMin=[]  DParamMax=[]  NParamMin=[]  NParamMax=[]  bParamMin=[]  bParamMax=[]  cParamMin=[]  cParamMax=[]  KbParamMin=[]  KbParamMax=[]  KtParamMin=[]  KtParamMax=[]  KbOutMin=[]  KbOutMax=[]  KtOutMin=[]  KtOutMax=[]  IntegratorOutMin=[]  IntegratorOutMax=[]  FilterOutMin=[]  FilterOutMax=[]  SumI1OutMin=[]  SumI1OutMax=[]  SumI2OutMin=[]  SumI2OutMax=[]  SumI3OutMin=[]  SumI3OutMax=[]  SumI4OutMin=[]  SumI4OutMax=[]  SumDOutMin=[]  SumDOutMax=[]  Sum1OutMin=[]  Sum1OutMax=[]  Sum2OutMin=[]  Sum2OutMax=[]  Sum3OutMin=[]  Sum3OutMax=[]  DifferentiatorOutMin=[]  DifferentiatorOutMax=[]  FilterDiffOutCoefMin=[]  FilterDiffOutCoefMax=[]  ReciprocalOutMin=[]  ReciprocalOutMax=[]  SumDenOutMin=[]  SumDenOutMax=[]  SumNumOutMin=[]  SumNumOutMax=[]  DivideOutMin=[]  DivideOutMax=[]  UdiffTsProdOutMin=[]  UdiffTsProdOutMax=[]  NTsProdOutMin=[]  NTsProdOutMax=[]  UintegralTsProdOutMin=[]  UintegralTsProdOutMax=[]  UngainTsProdOutMin=[]  UngainTsProdOutMax=[]  ClampingZeroOutDataTypeStr=Inherit: Inherit via back propagation  ClampingZeroOutMin=[]  ClampingZeroOutMax=[]  FilterDenConstantOutDataTypeStr=Inherit: Inherit via back propagation  FilterDenConstantOutMin=[]  FilterDenConstantOutMax=[]  PCopyOutDataTypeStr=Inherit: Inherit via back propagation  PCopyOutMin=[]  PCopyOutMax=[]  NCopyOutDataTypeStr=Inherit: Inherit via back propagation  NCopyOutMin=[]  NCopyOutMax=[]  IntegratorContinuousStateAttributes=''  IntegratorStateMustResolveToSignalObject=off  IntegratorRTWStateStorageClass=Auto  FilterContinuousStateAttributes=''  FilterStateMustResolveToSignalObject=off  FilterRTWStateStorageClass=Auto  ParallelPVariant=InternalParameters  IdealPVariant=Disabled  IVariant=InternalParameters  DVariant=InternalParameters  bVariant=InternalParameters  cVariant=InternalParameters  IntegratorVariant=Discrete  SatVariant=Disabled  AWVariant=Passthrough  PCopyVariant=Disabled  TRVariant=Disabled  FdbkBlocksVariant=Forward  IdealPFdbkVariant=Disabled  SatFdbkVariant=Disabled  DerivativeFilterVariant=ForwardEulerFilter  NVariant=InternalParameters  NCopyVariant=Disabled  FilterICVariant=InternalICsFilter  IntegratorICVariant=InternalICs  ExternalResetVariant=Disabled  TRSumVariant=Passthrough  SumFdbkVariant=Disabled  SumVariant=Sum_PID  TsampFilterVariant=InternalTs  TsampNgainVariant=Passthrough  TsampIntegralVariant=Disabled_SignalSpec  ExternalSaturationOutDataTypeStr=Inherit: Same as second input
      settings: LibrarySourceBlock=simulink/Discrete/Discrete PID Controller (2DOF)
  cfblk4 : DiscreteStateSpace
  cfblk5 : DiscreteStateSpace
  cfblk6 : DiscreteFilter  SampleTime=1
  cfblk7 : UnaryMinus
  cfblk8 : Reshape
  cfblk9 : Product  Inputs=**
  cfblk2 : Outport
  cfblk17 : Outport  Port=2
  wires:
  cfblk11/1 -> cfblk9/1
  cfblk9/1 -> cfblk8/1
  cfblk1/1 -> cfblk7/1
  cfblk4/1 -> cfblk10/1
  cfblk3/1 -> cfblk5/1
  cfblk12/1 -> cfblk4/1
  cfblk13/1 -> cfblk17/1
  cfblk14/1 -> cfblk6/1
  cfblk5/1 -> cfblk2/1
  cfblk6/1 -> cfblk10/2
  cfblk16/1 -> cfblk9/2
  cfblk7/1 -> cfblk10/3
  cfblk10/1 -> cfblk3/1
  cfblk8/1 -> cfblk3/2
